simulink model "comparaison_torque"  (R2020b)
settings: Solver=VariableStepAuto  StartTime=0.0  StopTime=10.0  RelTol=1e-3
settings Model: Creator=florian  LastModifiedBy=florian

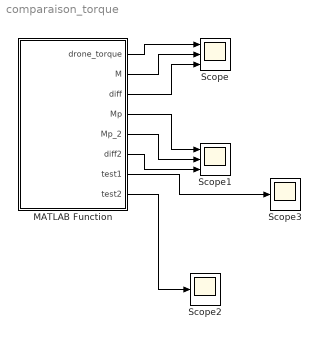
== system comparaison_torque ==
  MATLAB Function : MATLAB Function  TreatAsAtomicUnit=on
  Scope : Scope  NumInputPorts=3
  Scope1 : Scope  NumInputPorts=3
  Scope2 : Scope
  Scope3 : Scope
  wires:
  MATLAB Function/1(drone_torque) -> Scope/1
  MATLAB Function/2(M) -> Scope/2
  MATLAB Function/3(diff) -> Scope/3
  MATLAB Function/4(Mp) -> Scope1/1
  MATLAB Function/5(Mp_2) -> Scope1/2
  MATLAB Function/6(diff2) -> Scope1/3
  MATLAB Function/8(test2) -> Scope2/1
  MATLAB Function/7(test1) -> Scope3/1

== matlab function comparaison_torque/MATLAB Function ==
  data: drone_torque output; M output; diff output; Mp output; Mp_2 output; diff2 output; test1 output; test2 output
function [drone_torque, M, diff, Mp,Mp_2, diff2, test1, test2]= fcn()

drone = generateDarko();
p = [0;0;0];
v = [1;1;1];
q  = [1/sqrt(4);1/sqrt(4);1/sqrt(4);1/sqrt(4)];
w = [0;0;0];

x = [p;v;q;w];

T1 = 1.5;
T2 = 2.5;
d1 = deg2rad(-15);
d2 = deg2rad(15);

u = [T1;T2;d1; d2];
[~, Mp] = external_force_moment(x, u, 0, drone);

u_prime = [T1;T2;T1*d1; T2*d2];

% drone_torque = (drone.Mb*u_prime) + Mp;
 drone_torque = (drone.Mb*u_prime);

T1pT2 = T1+T2;
T1mT2 = T1-T2;
d1pd2 = d1+d2;
d1md2 = d1-d2;

D = q2dcm(q);

%% velocityin body frame
vb = D'*v;
vbx = vb(1);
vby = vb(2);
vbz = vb(3);

J = drone.INERTIA;


ay = drone.P_A2_CG(2);
py = drone.P_P2_CG(2);
die_c = drone.PHI(3,3);
Cd0 = drone.PHI(1,1);

Swet   = drone.WET_SURFACE;
Sdry   = drone.DRY_SURFACE;
Sp = pi*drone.PROP_RADIUS^2;
Thetam = drone.ELEVON_MEFFICIENCY(2);
Thetaf = drone.ELEVON_FEFFICIENCY(2);
kf = drone.PROP_KP;
km = drone.PROP_KM;
S = Swet + Sdry;
rho    = drone.RHO;
phi_n  = drone.PHI_n;
chord  = drone.CHORD;
ws     = drone.WINGSPAN;
B = diag([ws; chord; ws]);
dR = drone.CENTRAGE ;

eta = sqrt( norm(v)^2 + phi_n*norm(B*w)^2 );

% M = [
% (km/kf - (Swet/(8*Sp)) * ay * die_c * Thetaf *d1pd2)*T1mT2 + (-(Swet/(8*Sp))* ay * die_c * Thetaf* T1pT2 + 1/4 * rho* S * eta * ay * die_c * Thetaf* vbx)*d1md2; 
% (Swet/(8*Sp) * dR * die_c * Thetam * T1pT2 + 1/4 * rho* S * eta * dR * die_c * Thetam* vbx )* d1pd2 + Swet/(8*Sp) * dR * die_c * Thetam * T1mT2*d1md2 + 1/2 * rho* S *  dR  * die_c * eta *vbz ;
% -(py+Swet/(4*Sp)*ay*Cd0)*T1mT2 + (1/4 * rho* S * eta * ay * Cd0 * Thetaf* vbz)*d1md2
%     ];

M = [
(km/kf)*T1mT2 - (Swet/(8*Sp)) * ay * die_c * Thetaf * (d1pd2*T1mT2 + d1md2*T1pT2); 
(Swet/(8*Sp)) * dR * die_c * Thetam * (d1pd2*T1pT2 + d1md2*T1mT2) ;
-(py+Swet/(4*Sp)*ay*Cd0)*T1mT2 
    ];
test1 = -py*T1mT2;
test2 = Swet/(4*Sp)*ay*Cd0*T1mT2; 

Mp_2 = [
1/4 * rho* S * eta * ay * die_c * Thetaf* vbx * d1md2;
1/4 * rho* S * eta * dR * die_c * Thetam* vbx * d1pd2  + 1/2 * rho* S *  dR  * die_c * eta *vbz;
1/4 * rho* S * eta * ay * Cd0 * Thetaf* vbz * d1md2
];

diff = M-drone_torque;
diff2 = Mp_2-Mp;
